simulink model "project_589"  (R2020b)
settings: Solver=VariableStepAuto  StartTime=0.0  StopTime=2  RelTol=1e-3
libraries: powerlib x25, powerlib_meascontrol x8, simulink x7, re_lib x2, fillib x1
(part 1 of 2)
settings Model: Creator=mcapuano  LastModifiedBy=mcapuano
settings DebuggingCC: IgnoredZcDiagnostic=none

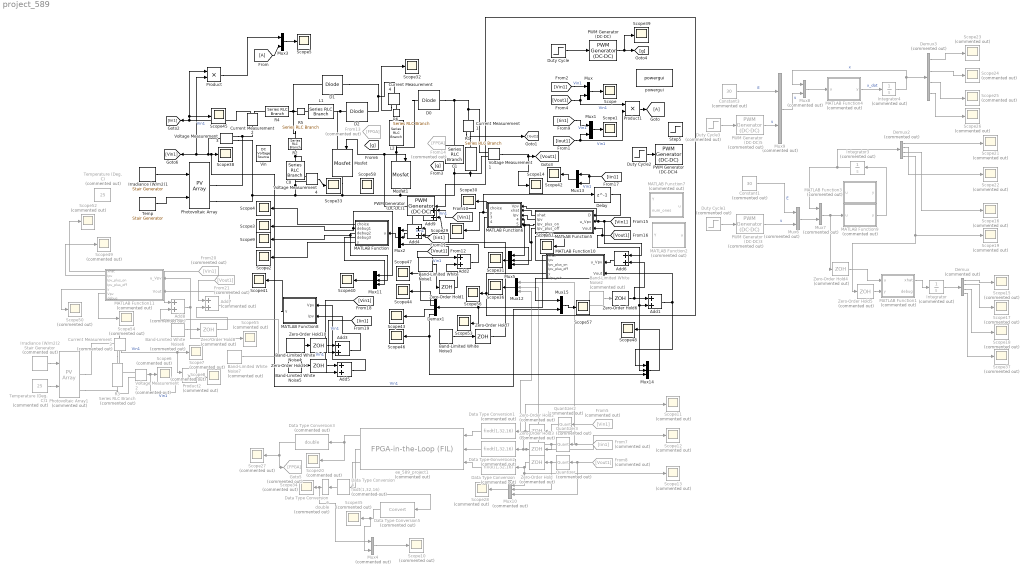
== system project_589 ==
  " Temp" : powerlib_meascontrol/Pulse & Signal Generators/Stair Generator  t=[0 .5 1 1.5]  e=[25 25 35 45]  Ts=15e-6
  Add{1..6,9} (7 alike) : Sum
  Add7 : Sum  Commented=on
  Add8 : Sum  Commented=on
  Band-Limited White Noise{1,3..5} (4 alike) : simulink/Sources/Band-Limited White Noise  Cov=[.0001]  Ts=1e-3  seed=[23341]
  Band-Limited White Noise2 : simulink/Sources/Band-Limited White Noise  Commented=on  Cov=[.00001]  Ts=15e-6  seed=[23341]
  Band-Limited White Noise6 : simulink/Sources/Band-Limited White Noise  Commented=on  Cov=[.0000001]  Ts=1e-6  seed=[23341]
  Band-Limited White Noise7 : simulink/Sources/Band-Limited White Noise  Commented=on  Cov=[.0000001]  Ts=15e-6  seed=[23341]
  C0 : powerlib/Elements/Series RLC Branch  LConnTagsString=__new0  RConnTagsString=__new0  BranchType=C  Resistance=1e-4  Inductance=200e-6  SetiL0=off  InitialCurrent=0  Capacitance=260e-6  Setx0=on  InitialVoltage=0  Measurements=None
  C1 : powerlib/Elements/Series RLC Branch  LConnTagsString=__new0  RConnTagsString=__new0  BranchType=C  Resistance=1e-4  Inductance=200e-6  SetiL0=off  InitialCurrent=0  Capacitance=260e-6  Setx0=on  InitialVoltage=0  Measurements=None
  Constant1 : Constant  Commented=on  Value=30
  Constant3 : Constant  Commented=on  Value=30
  Current Measurement1 : powerlib/Measurements/Current Measurement  PhasorSimulation=off  OutputType=Complex  PSBequivalent=0
  Current Measurement2 : powerlib/Measurements/Current Measurement  PhasorSimulation=off  OutputType=Complex  PSBequivalent=0
  Current Measurement3 : powerlib/Measurements/Current Measurement  Commented=on  PhasorSimulation=off  OutputType=Complex  PSBequivalent=0
  Current Measurement4 : powerlib/Measurements/Current Measurement  PhasorSimulation=off  OutputType=Complex  PSBequivalent=0
  D0 : powerlib/Power Electronics/Diode  Ron=1e-3  Lon=0  Vf=0  IC=0  UseSnubber=off  Rs=inf  Cs=inf  Measurements=off
  D1 : powerlib/Power Electronics/Diode  Ron=1e-3  Lon=0  Vf=0  IC=0  UseSnubber=off  Rs=inf  Cs=inf  Measurements=off
  D2 : powerlib/Power Electronics/Diode  Ron=1e-3  Lon=0  Vf=0  IC=0  UseSnubber=off  Rs=inf  Cs=inf  Measurements=off
  Data Type Conversion{,1..2,4} (4 alike) : DataTypeConversion  Commented=on  OutDataTypeStr=fixdt(1,32,16)
  Data Type Conversion3 : DataTypeConversion  Commented=on  OutDataTypeStr=double
  Data Type Conversion5 : DataTypeConversion  Commented=on
  Data Type Conversion6 : DataTypeConversion  Commented=on  OutDataTypeStr=double
  Delay : Delay  DelayLength=1  InitialCondition=0  SampleTime=15e-6
  Demux : Demux  Commented=on
  Demux1 : Demux
  Demux2 : Demux  Commented=on
  Demux3 : Demux  Commented=on
  Duty Cycle : Step  Time=.5  Before=.5  After=.5  SampleTime=0
  Duty Cycle1 : Step  Commented=on  Time=.5  Before=.5  After=.5  SampleTime=0
  Duty Cycle2 : Step  Time=.1  Before=.3  After=.5  SampleTime=0
  Duty Cycle3 : Step  Commented=on  Time=.5  Before=.5  After=.5  SampleTime=0
  From13 : From  Commented=on  GotoTag=FPGA
  From14 : From  Commented=on  GotoTag=FPGA
  From20 : From  Commented=on  GotoTag=Vin1
  From21 : From  Commented=on  GotoTag=Vout1
  From5 : From  Commented=on  GotoTag=Vin1
  From7 : From  Commented=on  GotoTag=Iin1
  From8 : From  Commented=on  GotoTag=Vout1
  Goto5 : Goto  Commented=on  GotoTag=FPGA
  Integrator : Integrator  Commented=on  InitialCondition=[0 0 0 0]
  Integrator3 : Integrator  Commented=on  InitialCondition=[0 0 0 0]
  Integrator4 : Integrator  Commented=on  InitialCondition=zeros(4,1)
  Irradiance (W/m2)1 : powerlib_meascontrol/Pulse & Signal Generators/Stair Generator  t=[0 .5]  e=[800 1000]  Ts=15e-6
  Irradiance (W/m2)2 : powerlib_meascontrol/Pulse & Signal Generators/Stair Generator  Commented=on  t=[0, 0.5, 1, 1.5, 2]  e=[0.5,0.7, 0.8, 0.6, 0.2]*1000  Ts=0.0001
  L1 : powerlib/Elements/Series RLC Branch  LConnTagsString=__new0  RConnTagsString=__new0  BranchType=L  Resistance=1e-4  Inductance=3e-3  SetiL0=on  InitialCurrent=0  Capacitance=30e-6  Setx0=off  InitialVoltage=150  Measurements=None
  L2 : powerlib/Elements/Series RLC Branch  LConnTagsString=__new0  RConnTagsString=__new0  BranchType=L  Resistance=1e-4  Inductance=3e-3  SetiL0=on  InitialCurrent=0  Capacitance=30e-6  Setx0=off  InitialVoltage=150  Measurements=None
  MATLAB Function : MATLAB Function  TreatAsAtomicUnit=on  SystemSampleTime=15e-6
  MATLAB Function1 : MATLAB Function  Commented=on  TreatAsAtomicUnit=on
  MATLAB Function10 : MATLAB Function  TreatAsAtomicUnit=on  SystemSampleTime=15e-6
  MATLAB Function11 : MATLAB Function  Commented=on  TreatAsAtomicUnit=on  SystemSampleTime=15e-6
  MATLAB Function2 : MATLAB Function  Commented=on  TreatAsAtomicUnit=on  SystemSampleTime=15e-6
  MATLAB Function3 : MATLAB Function  Commented=on  TreatAsAtomicUnit=on
  MATLAB Function4 : MATLAB Function  Commented=on  TreatAsAtomicUnit=on
  MATLAB Function5 : MATLAB Function  TreatAsAtomicUnit=on  SystemSampleTime=15e-6
  MATLAB Function6 : MATLAB Function  TreatAsAtomicUnit=on  SystemSampleTime=15e-6
  MATLAB Function7 : MATLAB Function  Commented=on  TreatAsAtomicUnit=on  SystemSampleTime=15e-6
  MATLAB Function8 : MATLAB Function  TreatAsAtomicUnit=on  SystemSampleTime=15e-6
  MATLAB Function9 : MATLAB Function  Commented=on  TreatAsAtomicUnit=on
  Mosfet : powerlib/Power Electronics/Mosfet  Ron=1e-3  Lon=0  Rd=1e-3  Vfd=0  IC=0  Rs=1e6  Cs=inf  Measurements=off
  Mosfet1 : powerlib/Power Electronics/Mosfet  Ron=1e-3  Lon=0  Rd=1e-3  Vfd=0  IC=0  Rs=1e6  Cs=inf  Measurements=off
  Mux{,1,3,13,15} (5 alike) : Mux  Inputs=2
  Mux10 : Mux  Commented=on  Inputs=3
  Mux{2,5,11..12,14} (5 alike) : Mux  Inputs=3
  Mux{4,6..9} (5 alike) : Mux  Commented=on  Inputs=2
  PWM Generator (DC-DC) : powerlib_meascontrol/Pulse & Signal Generators/PWM Generator (DC-DC)  Fsw=66.67e3  Ts=0
  PWM Generator (DC-DC)1 : powerlib_meascontrol/Pulse & Signal Generators/PWM Generator (DC-DC)  Fsw=66.67e3  Ts=0
  PWM Generator (DC-DC)3 : powerlib_meascontrol/Pulse & Signal Generators/PWM Generator (DC-DC)  Commented=on  Fsw=66.67e3  Ts=0
  PWM Generator (DC-DC)4 : powerlib_meascontrol/Pulse & Signal Generators/PWM Generator (DC-DC)  Fsw=66.67e3  Ts=0
  PWM Generator (DC-DC)5 : powerlib_meascontrol/Pulse & Signal Generators/PWM Generator (DC-DC)  Commented=on  Fsw=66.67e3  Ts=0
  Photovoltaic Array : re_lib/Solar/PV Array  Npar=1  Nser=1  PlotType=array @ 25 deg.C & specified irradiances  S_vec=[600 800 1000 1200]  Temp_C_vec=[25 50 75 100]  ModuleName=Kyocera Solar KC200GT  PlotWhenSelected=off  Pm=200.143  Ncell=54  Voc=32.9  Isc=8.21  Vm=26.3  Im=7.61  beta_Voc_pc=-0.355  alpha_Isc_pc=0.06  beta_Voc=-0.11679  alpha_Isc=0.004926  IL=8.2288  I0=2.3234e-10  nI=0.97734  Rsh=150.6844  Rs=0.34484  RobustModel=off  RobustCellTemperature=313.3991  BAL=on  Tc=1e-6  Tfilter=5e-5
      settings: AttributesFormatString=|
      | %<ModuleName>
      | %<Nser>-module string
      | %<Npar> parallel strings
  Photovoltaic Array1 : re_lib/Solar/PV Array  Commented=on  Npar=1  Nser=1  PlotType=one module @ 25 deg.C & specified irradiances  S_vec=[800]  Temp_C_vec=[ 50 ]  ModuleName=Kyocera Solar KC200GT  PlotWhenSelected=off  Pm=200.143  Ncell=54  Voc=32.9  Isc=8.21  Vm=26.3  Im=7.61  beta_Voc_pc=-0.355  alpha_Isc_pc=0.06  beta_Voc=-0.11679  alpha_Isc=0.004926  IL=8.2288  I0=2.3234e-10  nI=0.97734  Rsh=150.6844  Rs=0.34484  RobustModel=off  RobustCellTemperature=313.3991  BAL=on  Tc=1e-6  Tfilter=5e-5
      settings: AttributesFormatString=|
      | %<ModuleName>
      | %<Nser>-module string
      | %<Npar> parallel strings
  Product : Product
  Product1 : Product
  Product2 : Product  Commented=on
  Quantizer : Quantizer  Commented=on  QuantizationInterval=15e-6
  Quantizer2 : Quantizer  Commented=on  QuantizationInterval=15e-6
  Quantizer3 : Quantizer  Commented=on  QuantizationInterval=15e-6
  R1 : powerlib/Elements/Series RLC Branch  LConnTagsString=__new0  RConnTagsString=__new0  BranchType=R  Resistance=100  Inductance=200e-6  SetiL0=off  InitialCurrent=0  Capacitance=400e-6  Setx0=off  InitialVoltage=0  Measurements=None
  R2 : powerlib/Elements/Series RLC Branch  LConnTagsString=__new0  RConnTagsString=__new0  BranchType=R  Resistance=.01  Inductance=200e-6  SetiL0=off  InitialCurrent=0  Capacitance=400e-6  Setx0=off  InitialVoltage=0  Measurements=None
  R3 : powerlib/Elements/Series RLC Branch  Commented=on  LConnTagsString=__new0  RConnTagsString=__new0  BranchType=R  Resistance=1  Inductance=200e-6  SetiL0=off  InitialCurrent=0  Capacitance=400e-6  Setx0=off  InitialVoltage=0  Measurements=None
  R4 : powerlib/Elements/Series RLC Branch  LConnTagsString=__new0  RConnTagsString=__new0  BranchType=R  Resistance=.1  Inductance=200e-6  SetiL0=off  InitialCurrent=0  Capacitance=400e-6  Setx0=off  InitialVoltage=0  Measurements=None
  R5 : powerlib/Elements/Series RLC Branch  LConnTagsString=__new0  RConnTagsString=__new0  BranchType=R  Resistance=.0000001  Inductance=200e-6  SetiL0=off  InitialCurrent=0  Capacitance=400e-6  Setx0=off  InitialVoltage=0  Measurements=None
  R6 : powerlib/Elements/Series RLC Branch  LConnTagsString=__new0  RConnTagsString=__new0  BranchType=R  Resistance=.0000001  Inductance=200e-6  SetiL0=off  InitialCurrent=0  Capacitance=400e-6  Setx0=off  InitialVoltage=0  Measurements=None
  Scope{,1..5,9,14,29..33,36,38..48,51,53,56..58} (30 alike) : Scope
  Scope{6..8,10..13,15..28,34..35,37,49..50,52,54..55} (29 alike) : Scope  Commented=on
  Step5 : Step  Time=.1  Before=.1  After=.6  SampleTime=0
  Temperature (Deg. C) : Constant  Commented=on  Value=25
  Temperature (Deg. C)1 : Constant  Commented=on  Value=25
  Vin : powerlib/Electrical Sources/DC Voltage Source  Amplitude=30  Measurements=None
  Voltage Measurement1 : powerlib/Measurements/Voltage Measurement  PhasorSimulation=off  OutputType=Complex  PSBequivalent=0
  Voltage Measurement2 : powerlib/Measurements/Voltage Measurement  Commented=on  PhasorSimulation=off  OutputType=Complex  PSBequivalent=0
  Voltage Measurement3 : powerlib/Measurements/Voltage Measurement  PhasorSimulation=off  OutputType=Complex  PSBequivalent=0
  Voltage Measurement4 : powerlib/Measurements/Voltage Measurement  PhasorSimulation=off  OutputType=Complex  PSBequivalent=0
  Zero-Order Hold : ZeroOrderHold  Commented=on  SampleTime=200e-9
  Zero-Order Hold{1,6..7,10..11} (5 alike) : ZeroOrderHold  SampleTime=15e-6
  Zero-Order Hold2 : ZeroOrderHold  Commented=on  SampleTime=200e-9
  Zero-Order Hold3 : ZeroOrderHold  Commented=on  SampleTime=200e-9
  Zero-Order Hold4 : ZeroOrderHold  Commented=on  SampleTime=15e-6
  Zero-Order Hold5 : ZeroOrderHold  Commented=on  SampleTime=15e-6
  Zero-Order Hold8 : ZeroOrderHold  Commented=on  SampleTime=15e-6
  ee_589_project1 : fillib/FPGA-in-the-Loop (FIL)  Commented=on  ForceInterfaceUpdate=0.91338
      settings: SourceProductBaseCode=ES,HD
  powergui : powerlib/powergui  Priority=1  SimulationMode=Continuous  SampleTime=50e-6  frequency=60  Iterations=50  frequencyindice=0  Pbase=100e6  ErrMax=1e-4  UnitsV=kV  UnitsW=MW  buscounter=0  FunctionMessages=off  echomessages=off  EnableUseOfTLC=off  CurrentSourceSwitches=off  DisableSnubberDevices=off  DisableRonSwitches=off  DisableVfSwitches=off  DisplayEquations=off  AutomaticDiscreteSolvers=off  SolverType=Tustin/Backward Euler (TBE)  Interpol=off  ExternalGateDelay=off  methode=off  Ts=100  x0status=blocks  SPID=on  SwTol=0  HookPort=off  NonlinearTolerance=1e-4  nMaxIteration=100  ContinueOnMaxIteration=off  RestoreLinks=warning  ResistiveCurrentMeasurement=off  Frange=[0:2:500]  Ylog=off  Xlog=on  ShowGrid=off  save=off  variable=ZData  structure=0  ZoomFFT=off  StartTime=0.0  cycles=1  DisplayStyle=1  fundamental=60  FreqAxis=off  MaxFrequency=1000  frequencyindicesteady=1  RmsSteady=1  display=off
  wires:
  Duty Cycle/1 -> PWM Generator (DC-DC)/1
  PWM Generator (DC-DC)/1 -> Scope39/1, [g]
  Current Measurement1/1 -> [Iout1]
  Mux1/1 -> Scope1/1
  [Iout1] -> Product1/2, Mux1/2  "Vin1"
  [Iin1] -> Mux1/1  "Vin1"
  [Vin1] -> Mux/1  "Vin1"
  Mux/1 -> Scope/1
  [Vout1] -> Mux/2, Product1/1  "Vin1"
  Mux2/1 -> MATLAB Function/1(u)
  MATLAB Function/2(debug1) -> Scope3/1, Mux11/1
  MATLAB Function/1(choice) -> Scope4/1
  Voltage Measurement3/1 -> Product/2, [Vin1], Mux15/2, Scope38/1  "Vin1"
  Product/1 -> Mux3/1
  Current Measurement2/1 -> Scope45/1, Product/1, [Iin1]  "Vin1"
  Irradiance (W/m2)1/1 -> Photovoltaic Array/1
  Mux3/1 -> Scope5/1
  [A] -> Mux3/2
  Product1/1 -> [A]
  Temperature (Deg. C)1/1 -> Photovoltaic Array1/2
  Irradiance (W/m2)2/1 -> Photovoltaic Array1/1
  Voltage Measurement2/1 -> Product2/2, Scope6/1  "Vin1"
  Current Measurement3/1 -> Scope7/1, Product2/1  "Vin1"
  Product2/1 -> Scope8/1
  Constant1/1 -> Mux6/1  "E"
  Mux6/1 -> Mux7/2
  Mux7/1 -> MATLAB Function9/1(u), Zero-Order Hold4/1
  Demux2/3 -> Scope16/1
  Integrator3/1 -> Demux2/1, Mux7/1
  Demux2/2 -> Scope22/1
  Demux2/4 -> Scope19/1, Zero-Order Hold5/1
  Demux2/1 -> Scope21/1
  PWM Generator (DC-DC)3/1 -> Mux6/2  "u"
  Duty Cycle1/1 -> PWM Generator (DC-DC)3/1
  Integrator4/1 -> Mux8/1, Demux3/1  "x"
  Constant3/1 -> Mux9/1  "E"
  Mux9/1 -> Mux8/2  "u"
  MATLAB Function4/1(y) -> Integrator4/1  "x_dot"
  Demux3/2 -> Scope24/1
  Demux3/1 -> Scope23/1
  Mux8/1 -> MATLAB Function4/1(u)
  Demux3/3 -> Scope25/1
  Demux3/4 -> Scope26/1
  Duty Cycle2/1 -> PWM Generator (DC-DC)4/1
  Mux10/1 -> Scope28/1
  Quantizer/1 -> Mux10/2, Zero-Order Hold/1
  Zero-Order Hold/1 -> Mux10/1, Scope13/1, Data Type Conversion/1
  Current Measurement4/1 -> Scope32/1
  Data Type Conversion2/1 -> ee_589_project1/2
  Data Type Conversion1/1 -> ee_589_project1/1
  Zero-Order Hold2/1 -> Scope11/1, Data Type Conversion1/1
  Zero-Order Hold3/1 -> Data Type Conversion2/1, Mux12/3, Scope12/1
  Quantizer3/1 -> Mux12/2, Zero-Order Hold3/1
  Quantizer2/1 -> Zero-Order Hold2/1
  From5/1 -> Quantizer2/1
  From7/1 -> Mux12/1, Quantizer3/1
  From8/1 -> Mux10/3, Quantizer/1
  Data Type Conversion5/1 -> Mux4/2, Scope35/1
  ee_589_project1/3 -> Data Type Conversion5/1
  Mux12/1 -> Scope36/1
  Data Type Conversion4/1 -> Data Type Conversion6/1
  Data Type Conversion3/1 -> Goto5/1, Scope27/1
  ee_589_project1/1 -> Data Type Conversion3/1, Scope20/1
  ee_589_project1/2 -> Data Type Conversion4/1
  Data Type Conversion6/1 -> Mux4/1, Scope34/1
  Data Type Conversion/1 -> ee_589_project1/3
  MATLAB Function/3(debug2) -> Mux11/2, Scope9/1
  Mux4/1 -> Scope10/1
  Demux/1 -> Scope15/1
  Demux/2 -> Scope17/1
  Demux/3 -> Scope18/1
  Demux/4 -> Scope37/1
  MATLAB Function1/1(xhat) -> Integrator/1
  Integrator/1 -> Demux/1
  Zero-Order Hold4/1 -> MATLAB Function1/1(u)
  Zero-Order Hold5/1 -> MATLAB Function1/2(y)
  MATLAB Function/5(y) -> Scope2/1
  [Vin1] -> Add6/1, MATLAB Function6/1(Vpv), MATLAB Function5/2(u_Vpv)
  [Vout1] -> Mux14/2, Add1/2, MATLAB Function5/3(Vout)
  MATLAB Function5/1(xhat) -> MATLAB Function6/2(xhat)
  MATLAB Function5/3(Ipv_plus_on) -> Mux5/1, MATLAB Function6/4(Ipv_plus_on)
  MATLAB Function5/4(Ipv_plus_off) -> Mux5/2, MATLAB Function6/5(Ipv_plus_off)
  MATLAB Function6/2(y) -> Delay/1, Scope29/1
  MATLAB Function6/1(choice) -> Scope30/1
  Mux5/1 -> Scope31/1
  Mux11/1 -> Scope40/1
  MATLAB Function/4(debug3) -> Mux11/3
  Mux13/1 -> Scope42/1
  [Iin1] -> Mux13/2, Mux13/1  "Vin1"
  Demux1/1 -> Scope47/1
  Demux1/2 -> Scope44/1
  Demux1/3 -> Scope43/1
  Demux1/4 -> Mux14/3, Scope46/1
  MATLAB Function6/3(debug1) -> Mux5/3
  MATLAB Function5/2(Ipv) -> MATLAB Function6/3(Ipv)
  MATLAB Function8/1(Y) -> Scope41/1
  Duty Cycle3/1 -> PWM Generator (DC-DC)5/1
  PWM Generator (DC-DC)5/1 -> Mux9/2  "u"
  MATLAB Function9/1(y) -> Integrator3/1
  Voltage Measurement4/1 -> Scope33/1
  Delay/1 -> MATLAB Function5/1(D)
  " Temp"/1 -> Photovoltaic Array/2
  Voltage Measurement1/1 -> Scope14/1, [Vout1]
  Band-Limited White Noise2/1 -> Zero-Order Hold6/1
  Zero-Order Hold6/1 -> Add6/2, Add1/1
  Add1/1 -> Mux14/1, MATLAB Function10/2(Vout)
  Zero-Order Hold1/1 -> Add2/2
  [Vout1] -> Add2/1  "Vin1"
  Add2/1 -> Mux2/3
  Band-Limited White Noise1/1 -> Zero-Order Hold1/1
  Add4/1 -> Mux2/2
  [Iin1] -> Add4/1  "Vin1"
  [Iin1] -> Add3/2  "Vin1"
  [Vin1] -> Add5/2  "Vin1"
  Add5/1 -> MATLAB Function8/1(Vpv)
  Add3/1 -> MATLAB Function8/2(Ipv)
  Zero-Order Hold7/1 -> Add4/2, Add9/2
  Band-Limited White Noise3/1 -> Zero-Order Hold7/1
  Mux14/1 -> Scope48/1
  Add6/1 -> MATLAB Function10/1(u_Vpv)
  MATLAB Function11/2(Ipv) -> Scope49/1
  MATLAB Function10/2(Ipv) -> Scope51/1
  MATLAB Function11/1(xhat) -> Scope52/1
  MATLAB Function10/1(xhat) -> Scope53/1, Demux1/1
  MATLAB Function11/6(Vpv) -> Scope54/1
  MATLAB Function10/5(y) -> PWM Generator (DC-DC)1/1, Scope56/1
  MATLAB Function11/5(y) -> Scope50/1
  Band-Limited White Noise6/1 -> Zero-Order Hold8/1
  Zero-Order Hold8/1 -> Add7/2
  From21/1 -> Add7/1
  Add7/1 -> MATLAB Function11/2(Vout)
  From20/1 -> Add8/1
  Add8/1 -> MATLAB Function11/1(u_Vpv), Scope55/1
  Band-Limited White Noise7/1 -> Add8/2
  Band-Limited White Noise4/1 -> Zero-Order Hold10/1
  Zero-Order Hold10/1 -> Add3/1
  Band-Limited White Noise5/1 -> Zero-Order Hold11/1
  Zero-Order Hold11/1 -> Add5/1
  [Vin1] -> Add9/1  "Vin1"
  Add9/1 -> Mux2/1
  PWM Generator (DC-DC)1/1 -> Mosfet/1, Mosfet1/1
  Mux15/1 -> Scope57/1
  MATLAB Function10/6(Vpv_out) -> Mux15/1
  connections:
  D0/RConn1 -- C1/LConn1 -- Current Measurement1/LConn1 -- Voltage Measurement1/LConn1
  R2/LConn1 -- R5/LConn1 -- R4/RConn1 -- D1/LConn1
  C1/RConn1 -- Mosfet/RConn1 -- Voltage Measurement3/LConn2 -- Photovoltaic Array/RConn2 -- Voltage Measurement4/LConn2 -- C0/RConn1 -- Mosfet1/RConn1 -- Voltage Measurement1/LConn2 -- R1/RConn1
  Mosfet/LConn1 -- L1/RConn1 -- D2/LConn1
  D1/RConn1 -- Current Measurement4/LConn1 -- D2/RConn1
  D0/LConn1 -- Mosfet1/LConn1 -- L2/RConn1
  Current Measurement1/RConn1 -- R1/LConn1
  R2/RConn1 -- Voltage Measurement4/LConn1 -- C0/LConn1
  Voltage Measurement3/LConn1 -- Current Measurement2/LConn1 -- Photovoltaic Array/RConn1
  Photovoltaic Array1/RConn1 -- Current Measurement3/LConn1 -- Voltage Measurement2/LConn1
  Photovoltaic Array1/RConn2 -- Voltage Measurement2/LConn2 -- R3/RConn1
  Current Measurement3/RConn1 -- R3/LConn1
  R4/LConn1 -- Current Measurement2/RConn1
  R5/RConn1 -- L1/LConn1
  R6/LConn1 -- Current Measurement4/RConn1
  R6/RConn1 -- L2/LConn1

== matlab function project_589/MATLAB Function9 ==
  data: u input; y output
function y = fcn(u)

X=u(1:4);
Vpv=u(5);
u=u(6);



% parameters:
%5/10/2021 u_ePDATED


Cpv=260e-6;
Cout=260e-6;
L1=3e-3;
L2=3e-3;
Rout=100;
Rpv = 1;
RL1 = 1;
RL2 = 1;

u_e = .5;

% Compact form
A=[(-1/(Cpv*Rpv)) (-1/(Cpv)) (-u_e/(Cpv)) 0 ;
    (1/(L1+L2) + L2*u_e/(L1*(L1+L2)))  (-RL1/(L1+L2) -RL1*L2*u_e/(L1*(L1+L2)))  (-RL2/(L1+L2) + RL2*u_e/(L1+L2)) (-1/(L1+L2) + u_e/(L1+L2));
    (1/(L1+L2) + L1*u_e/(L2*(L1+L2)))  (-RL1/(L1+L2) + RL1*u_e/(L1+L2)) (-RL2/(L1+L2)-RL2*L1*u_e/(L2*(L1+L2))) (-1/(L1+L2) + u_e/(L1+L2));
    0 0 (1/(Cout) - u_e/(Cout)) (-1/(Rout*Cout))];

%VCpv = (L2*RL1*Rout*Vpv*u_e^2 - 2*L2*RL1*Rout*Vpv*u_e + L1*RL1*RL2*Vpv + L2*RL1*RL2*Vpv + L2*RL1*Rout*Vpv)/(L1*RL1*RL2 + L2*RL1*RL2 + L2*RL1*Rout + L2*RL2*Rpv - L1*Rout*Rpv + L2*Rout*Rpv + L2*RL1*Rout*u_e^2 + L2*RL1*Rpv*u_e^2 - L1*Rout*Rpv*u_e^2 + L2*Rout*Rpv*u_e^2 - 2*L2*RL1*Rout*u_e + L1*RL1*Rpv*u_e + L1*RL2*Rpv*u_e + 2*L1*Rout*Rpv*u_e - 2*L2*Rout*Rpv*u_e);
%IL1 = (Vpv*(L2*RL2 - L1*Rout + L2*Rout + L1*RL2*u_e + 2*L1*Rout*u_e - 2*L2*Rout*u_e - L1*Rout*u_e^2 + L2*Rout*u_e^2))/(L1*RL1*RL2 + L2*RL1*RL2 + L2*RL1*Rout + L2*RL2*Rpv - L1*Rout*Rpv + L2*Rout*Rpv + L2*RL1*Rout*u_e^2 + L2*RL1*Rpv*u_e^2 - L1*Rout*Rpv*u_e^2 + L2*Rout*Rpv*u_e^2 - 2*L2*RL1*Rout*u_e + L1*RL1*Rpv*u_e + L1*RL2*Rpv*u_e + 2*L1*Rout*Rpv*u_e - 2*L2*Rout*Rpv*u_e);
%IL2 = (RL1*Vpv*(L1 + L2*u_e))/(L1*RL1*RL2 + L2*RL1*RL2 + L2*RL1*Rout + L2*RL2*Rpv - L1*Rout*Rpv + L2*Rout*Rpv + L2*RL1*Rout*u_e^2 + L2*RL1*Rpv*u_e^2 - L1*Rout*Rpv*u_e^2 + L2*Rout*Rpv*u_e^2 - 2*L2*RL1*Rout*u_e + L1*RL1*Rpv*u_e + L1*RL2*Rpv*u_e + 2*L1*Rout*Rpv*u_e - 2*L2*Rout*Rpv*u_e);
%VCout = -(RL1*Rout*Vpv*(L1 + L2*u_e)*(u_e - 1))/(L1*RL1*RL2 + L2*RL1*RL2 + L2*RL1*Rout + L2*RL2*Rpv - L1*Rout*Rpv + L2*Rout*Rpv + L2*RL1*Rout*u_e^2 + L2*RL1*Rpv*u_e^2 - L1*Rout*Rpv*u_e^2 + L2*Rout*Rpv*u_e^2 - 2*L2*RL1*Rout*u_e + L1*RL1*Rpv*u_e + L1*RL2*Rpv*u_e + 2*L1*Rout*Rpv*u_e - 2*L2*Rout*Rpv*u_e);

VCpv = (L2*RL1*Rout*Vpv*u_e^2 - 2*L2*RL1*Rout*Vpv*u_e + L1*RL1*RL2*Vpv + L2*RL1*RL2*Vpv + L2*RL1*Rout*Vpv)/(L1*RL1*RL2 + L2*RL1*RL2 + L2*RL1*Rout + L2*RL2*Rpv - L1*Rout*Rpv + L2*Rout*Rpv + L2*RL1*Rout*u_e^2 + L2*RL1*Rpv*u_e^2 - L1*Rout*Rpv*u_e^2 + L2*Rout*Rpv*u_e^2 - 2*L2*RL1*Rout*u_e + L1*RL1*Rpv*u_e + L1*RL2*Rpv*u_e + 2*L1*Rout*Rpv*u_e - 2*L2*Rout*Rpv*u_e);
IL1 = (Vpv*(L2*RL2 - L1*Rout + L2*Rout + L1*RL2*u_e + 2*L1*Rout*u_e - 2*L2*Rout*u_e - L1*Rout*u_e^2 + L2*Rout*u_e^2))/(L1*RL1*RL2 + L2*RL1*RL2 + L2*RL1*Rout + L2*RL2*Rpv - L1*Rout*Rpv + L2*Rout*Rpv + L2*RL1*Rout*u_e^2 + L2*RL1*Rpv*u_e^2 - L1*Rout*Rpv*u_e^2 + L2*Rout*Rpv*u_e^2 - 2*L2*RL1*Rout*u_e + L1*RL1*Rpv*u_e + L1*RL2*Rpv*u_e + 2*L1*Rout*Rpv*u_e - 2*L2*Rout*Rpv*u_e);
IL2 =  (RL1*Vpv*(L1 + L2*u_e))/(L1*RL1*RL2 + L2*RL1*RL2 + L2*RL1*Rout + L2*RL2*Rpv - L1*Rout*Rpv + L2*Rout*Rpv + L2*RL1*Rout*u_e^2 + L2*RL1*Rpv*u_e^2 - L1*Rout*Rpv*u_e^2 + L2*Rout*Rpv*u_e^2 - 2*L2*RL1*Rout*u_e + L1*RL1*Rpv*u_e + L1*RL2*Rpv*u_e + 2*L1*Rout*Rpv*u_e - 2*L2*Rout*Rpv*u_e);
VCout =  -(RL1*Rout*Vpv*(L1 + L2*u_e)*(u_e - 1))/(L1*RL1*RL2 + L2*RL1*RL2 + L2*RL1*Rout + L2*RL2*Rpv - L1*Rout*Rpv + L2*Rout*Rpv + L2*RL1*Rout*u_e^2 + L2*RL1*Rpv*u_e^2 - L1*Rout*Rpv*u_e^2 + L2*Rout*Rpv*u_e^2 - 2*L2*RL1*Rout*u_e + L1*RL1*Rpv*u_e + L1*RL2*Rpv*u_e + 2*L1*Rout*Rpv*u_e - 2*L2*Rout*Rpv*u_e);
 
B=[ -IL2/Cpv;
    L2*VCpv/(L1*(L1+L2))-RL1*L2*IL1/(L1*(L1+L2))+RL2*IL2/(L1+L2)+VCout/(L1+L2);
    L1*VCpv/(L2*(L1+L2))+RL1*IL1/(L1+L2)-RL2*L1*IL2/(L2*(L1+L2))+VCout/(L1+L2);
     -IL2/Cout];


% B = [1/(Cpv*Rpv);
%     0;
%     0;
%     0];

%u = Vpv;

y = A*X+B*u;

== matlab function project_589/MATLAB Function10 ==
  data: xhat output; u_Vpv input; Vout input; Ipv output; Ipv_plus_on output; Ipv_plus_off output; y output; Vpv_out output
function [xhat, Ipv, Ipv_plus_on, Ipv_plus_off, y, Vpv_out]  = fcn(u_Vpv, Vout)
%Kalman filter design using Small Signal Model of Circuit

%The purpose of this module is to approximate Ipv and Vpv so that a sensor
%is not needed for those variables, it also functions to remove noise and
%could possibly replace the MCP module using its own predictions

%Existing Model assumes Constant Vpv with added series resistor so that
% Ipv = (Vpv - Vcpv)/Rpv
%Also assumes L1 = L2

%Existing state variables: IL1 IL2 Vo Vcpv

%define circuit parameters 


Cpv=260e-6;
Cout=260e-6;
L1=3e-3;
L2=3e-3;
Rout=100;
Rpv = .1;
RL1 = .0000001;
RL2 = .0000001;

persistent Est_Vpv;
if isempty(Est_Vpv)
    Est_Vpv = 0;
end
persistent DC;
if isempty(DC)
    DC = 0;
end
Vpv = u_Vpv;
y = Vout;
u = u_Vpv;

Ts = 15e-6;
% Continuous Time Small Signal State Space
%Aol = [0.943784461257301,-0.0559330122345799,-0.0279395312339836,5.29606701473712e-05;0.00363447688363775,0.996152021590196,-0.00131615408875196,-0.00124644633684318;0.00363447688363775,-0.00135110080726459,0.996186968308708,-0.00124644633684318;5.29606701473712e-05,-1.90030480999995e-05,0.0287831492829427,0.999405251934562];
Ac =[(-1/(Cpv*Rpv)) (-1/(Cpv)) (-DC/(Cpv)) 0 ;
    (1/(L1+L2) + L2*DC/(L1*(L1+L2)))  (-RL1/(L1+L2) -RL1*L2*DC/(L1*(L1+L2)))  (-RL2/(L1+L2) + RL2*DC/(L1+L2)) (-1/(L1+L2) + DC/(L1+L2));
    (1/(L1+L2) + L1*DC/(L2*(L1+L2)))  (-RL1/(L1+L2) + RL1*DC/(L1+L2)) (-RL2/(L1+L2)-RL2*L1*DC/(L2*(L1+L2))) (-1/(L1+L2) + DC/(L1+L2));
    0 0 (1/(Cout) - DC/(Cout)) (-1/(Rout*Cout))];
Bc = [1/(Cpv*Rpv);
    0;
    0;
    0];
 Cc = [0 0 0 1];
 
 Dc = zeros(size(Cc,1), size(Bc,2));
 
 %discretize my state space model using ZOH method
 Aol = eye(4) + Ac*Ts;
 Bol = Bc*Ts;
 Col = Cc;
 Dol = Dc;
 
 
%Bol = [0.0560566260169120;0.000105941817191590;0.000105941817191590;1.02384484238660e-06];

%Col = [0,0,0,1];

%Dol = 0;
 %Design the Observer System:
 

 %covar matricies, process q, measurement r -- must be positive numbers
 Qcov = diag(.000000001*ones(1,4)); %modify the numbers to change how it filters noise
 Rcov = diag(.01*ones(1,1)); %modify the numbers to change how it filters noise
 

persistent xhat_t_1; %previous xhat Sample
if isempty(xhat_t_1)
    xhat_t_1 = [.1; .1; .1; .1];
end

persistent P_t_1;
if isempty(P_t_1)
    P_t_1 = [.1 .1 .1 .1;
            .1 .1 .1 .1;
            .1 .1 .1 .1;
            .1 .1 .1 .1];
end


%prediction stage
xhat_pred = Aol*xhat_t_1+Bol*u;
P_pred = Aol*P_t_1*transpose(Aol)+ Qcov;

%update stage
y_update = y - Col*xhat_pred;
S_update = Col*P_pred*transpose(Col) + Rcov;
K_update = P_pred*transpose(Col)*(1/S_update);
xhat_update = xhat_pred + K_update*y_update;
P_update = (eye(4) - K_update*Col)*P_pred;

Est_Vpv =  xhat_update(4)*(1-DC)/(1+DC) + .35;
 Vpv_out = Est_Vpv;

%increase DC by .01:
DC = DC + .0001;
if(DC > 1)
    DC = 1;
end
Ac =[(-1/(Cpv*Rpv)) (-1/(Cpv)) (-DC/(Cpv)) 0 ;
    (1/(L1+L2) + L2*DC/(L1*(L1+L2)))  (-RL1/(L1+L2) -RL1*L2*DC/(L1*(L1+L2)))  (-RL2/(L1+L2) + RL2*DC/(L1+L2)) (-1/(L1+L2) + DC/(L1+L2));
    (1/(L1+L2) + L1*DC/(L2*(L1+L2)))  (-RL1/(L1+L2) + RL1*DC/(L1+L2)) (-RL2/(L1+L2)-RL2*L1*DC/(L2*(L1+L2))) (-1/(L1+L2) + DC/(L1+L2));
    0 0 (1/(Cout) - DC/(Cout)) (-1/(Rout*Cout))];
Aol_increase = eye(4) + Ac*Ts;
%predict 1 timestep ahead on
xhat_plus_on = Aol_increase*xhat_update + Bol*u;
Ipv_plus_on = (u - xhat_plus_on(1))/Rpv;
%decrease DC by .01
DC = DC - 2*.0001;
if(DC < 0) 
    DC = 0; end
Ac =[(-1/(Cpv*Rpv)) (-1/(Cpv)) (-DC/(Cpv)) 0 ;
    (1/(L1+L2) + L2*DC/(L1*(L1+L2)))  (-RL1/(L1+L2) -RL1*L2*DC/(L1*(L1+L2)))  (-RL2/(L1+L2) + RL2*DC/(L1+L2)) (-1/(L1+L2) + DC/(L1+L2));
    (1/(L1+L2) + L1*DC/(L2*(L1+L2)))  (-RL1/(L1+L2) + RL1*DC/(L1+L2)) (-RL2/(L1+L2)-RL2*L1*DC/(L2*(L1+L2))) (-1/(L1+L2) + DC/(L1+L2));
    0 0 (1/(Cout) - DC/(Cout)) (-1/(Rout*Cout))];
DC = DC + .0001;
Aol_decrease = eye(4) + Ac*Ts;
%predict 1 timestep ahead off
xhat_plus_off = Aol_decrease*xhat_update + Bol*u;
Ipv_plus_off = (u - xhat_plus_off(1))/Rpv;

%update function output and variables
P_t_1 = P_update;
xhat_t_1 = xhat_update;
xhat = xhat_update;
Ipv = (u - xhat(1))/Rpv;

%%%%%%%%%%%%%%%%%%%%%%%%%%%%%%%
if (Ipv > 10)
    Ipv = 1;
end



persistent Vpv_t_1; %previous Vpv Sample
if isempty(Vpv_t_1)
    Vpv_t_1 = 0;
end
persistent Ipv_t_1; %previous Ipv Sample
if isempty(Ipv_t_1)
    Ipv_t_1 = 0;
end
persistent Dpv_t_1; % Iref (output) value from what is now 2 timesteps ago
if isempty(Dpv_t_1)
    Dpv_t_1 = 0;
end
persistent Dpv;  %Previous / Most recent Iref (output) Calc
if isempty(Dpv)
    Dpv = 0;
end

Ts = 15e-6; %sample rate
L = 3e-3; %inductance


delta_V = Vpv - Vpv_t_1;
delta_I = Ipv - Ipv_t_1;
delta_D = Dpv - Dpv_t_1;


%fixed vs adaptive
scale_factor_C = 10; %increase for larger output increments/swings
 Z =.001; %fixed 
%Z = scale_factor_C * abs(delta_I * delta_D); %adaptive

% custom adaptive to fix issues with no change causing 0 step size
 adapZ = scale_factor_C * abs(delta_I * delta_D);
% if(adapZ > .1)
%     Z = .1;
% elseif(adapZ > .001)
%     Z = adapZ;
% else
%     Z = .001;
% end

Ipred_1 = Ipv_plus_on;
Ipred_0 = Ipv_plus_off;
%Ipred_1 = Ipv + 2*(Ts/L) * Vpv; %MPC prediction for switch = 1
%Ipred_0 = Ipv + (Ts/(2*L)* (Vpv - Vout)); %MPC prediction for switch = 0 

if delta_V == 0 %Inc. Cond. Algo to determine Iref
    if delta_I == 0 
        Iref = Dpv; choice = 0;
    else
        if delta_I > 0
            Iref = Dpv - Z; choice = 1;
        else
            Iref = Dpv + Z; choice = 2;
        end
    end
else
    if (Ipv + (delta_I/delta_V) * Vpv) == 0
        Iref = Dpv; choice = 3;
    else
        if (Ipv + (delta_I/delta_V) * Vpv) > 0
            Iref = Dpv - Z; choice = 4;
        else
            Iref = Dpv + Z; choice = 5;
        end
    end
end

G1 = abs(Iref - Ipred_1); %Optimize MPC by applying Iref
G0 = abs(Iref - Ipred_0);
if G1 < G0
    DC = DC + .0001;
else
    DC = DC - .0001;
end

if (DC < 0)
    DC = 0;
end
if (DC > 1)
    DC = 1;
end

if (Iref < 0)
    Iref = .001;
end
%test = Ipv + (delta_I/delta_V) * Vpv;
test =  delta_V;
%update static variables here:
Vpv_t_1 = Vpv; %previous Vpv Sample
Ipv_t_1 = Ipv; %previous Ipv Sample
Dpv_t_1 = Dpv; % Iref (output) value from what is now 2 timesteps ago
Dpv = Iref;  %Previous / Most recent Iref (output) Calc

y = DC;

%debug purposes:
debug1 = Iref;
debug2 = delta_I/delta_V;

== matlab function project_589/MATLAB Function11 ==
  data: xhat output; u_Vpv input; Vout input; Ipv output; Ipv_plus_on output; Ipv_plus_off output; y output; Vpv output; debug output
function [xhat, Ipv, Ipv_plus_on, Ipv_plus_off, y, Vpv, debug]  = fcn(u_Vpv, Vout)
%Kalman filter design using Small Signal Model of Circuit

%The purpose of this module is to approximate Ipv and Vpv so that a sensor
%is not needed for those variables, it also functions to remove noise and
%could possibly replace the MCP module using its own predictions

%Existing Model assumes Constant Vpv with added series resistor so that
% Ipv = (Vpv - Vcpv)/Rpv
%Also assumes L1 = L2

%Existing state variables: IL1 IL2 Vo Vcpv

%define circuit parameters 


Cpv=260e-6;
Cout=260e-6;
L1=3e-3;
L2=3e-3;
Rout=100;
Rpv = 1;
RL1 = 1;
RL2 = 1;
persistent DC;
if isempty(DC)
    DC = 0;
end

y = Vout;
u = u_Vpv;

Ts = 15e-6;
% Continuous Time Small Signal State Space
%Aol = [0.943784461257301,-0.0559330122345799,-0.0279395312339836,5.29606701473712e-05;0.00363447688363775,0.996152021590196,-0.00131615408875196,-0.00124644633684318;0.00363447688363775,-0.00135110080726459,0.996186968308708,-0.00124644633684318;5.29606701473712e-05,-1.90030480999995e-05,0.0287831492829427,0.999405251934562];
Ac =[(-1/(Cpv*Rpv)) (-1/(Cpv)) (-DC/(Cpv)) 0 ;
    (1/(L1+L2) + L2*DC/(L1*(L1+L2)))  (-RL1/(L1+L2) -RL1*L2*DC/(L1*(L1+L2)))  (-RL2/(L1+L2) + RL2*DC/(L1+L2)) (-1/(L1+L2) + DC/(L1+L2));
    (1/(L1+L2) + L1*DC/(L2*(L1+L2)))  (-RL1/(L1+L2) + RL1*DC/(L1+L2)) (-RL2/(L1+L2)-RL2*L1*DC/(L2*(L1+L2))) (-1/(L1+L2) + DC/(L1+L2));
    0 0 (1/(Cout) - DC/(Cout)) (-1/(Rout*Cout))];
Bc = [1/(Cpv*Rpv);
    0;
    0;
    0];
 Cc = [0 0 0 1];
 
 Dc = zeros(size(Cc,1), size(Bc,2));
 
 %discretize my state space model using ZOH method
 Aol = eye(4) + Ac*Ts;
 Bol = Bc*Ts;
 Col = Cc;
 Dol = Dc;
 
 
%Bol = [0.0560566260169120;0.000105941817191590;0.000105941817191590;1.02384484238660e-06];

%Col = [0,0,0,1];

%Dol = 0;
 %Design the Observer System:
 

 %covar matricies, process q, measurement r -- must be positive numbers
 Qcov = diag(1*ones(1,4)); %modify the numbers to change how it filters noise
 Rcov = diag(1*ones(1,1)); %modify the numbers to change how it filters noise
 
variance = 1;
persistent xhat_t_1; %previous xhat Sample
if isempty(xhat_t_1)
    xhat_t_1 = [.1; .1; .1; .1];
end

persistent P_t_1;
if isempty(P_t_1)
    P_t_1 = [.1 .1 .1 .1 ;
            .1 .1 .1 .1 ;
            .1 .1 .1 .1 ;
            .1 .1 .1 .1 ];
end


%prediction stage
xhat_pred = Aol*xhat_t_1+Bol*u;
P_pred = Aol*P_t_1*transpose(Aol)+ variance*Bol*transpose(Bol) + Qcov;

%update stage
y_update = y - Col*xhat_pred;
S_update = Col*P_pred*transpose(Col) + Rcov - variance;
K_update = P_pred*transpose(Col)*(1/S_update);
xhat_update = xhat_pred + K_update*y_update;
P_update = (eye(4) - K_update*Col)*P_pred;


    Ipv1 = xhat_update(2) + xhat_update(3) + Cpv*((xhat_update(1) - xhat_t_1(1)) / Ts); debug = 1;
 
    Ipv0 = xhat_update(2) + Cpv*((xhat_update(1) - xhat_t_1(1)) / Ts); debug = 0;

    Ipv = (Ipv1*DC + Ipv0*(1-DC));

    if(Ipv < 0)
        Ipv = 0;
    end
    
u = Ipv * Rpv + xhat_update(1);
%Ipv = (u - xhat(1))/Rpv;

%increase DC by .01:
DC = DC + .0001;
if(DC > 1)
    DC = 1;
end
Ac =[(-1/(Cpv*Rpv)) (-1/(Cpv)) (-DC/(Cpv)) 0 ;
    (1/(L1+L2) + L2*DC/(L1*(L1+L2)))  (-RL1/(L1+L2) -RL1*L2*DC/(L1*(L1+L2)))  (-RL2/(L1+L2) + RL2*DC/(L1+L2)) (-1/(L1+L2) + DC/(L1+L2));
    (1/(L1+L2) + L1*DC/(L2*(L1+L2)))  (-RL1/(L1+L2) + RL1*DC/(L1+L2)) (-RL2/(L1+L2)-RL2*L1*DC/(L2*(L1+L2))) (-1/(L1+L2) + DC/(L1+L2));
    0 0 (1/(Cout) - DC/(Cout)) (-1/(Rout*Cout))];
Aol_increase = eye(4) + Ac*Ts;
%predict 1 timestep ahead on
xhat_plus_on = Aol_increase*xhat_update + Bol*u;
Ipv_plus_on = (u - xhat_plus_on(1))/Rpv;
%decrease DC by .01
DC = DC - 2*.0001;
if(DC < 0) 
    DC = 0; end
Ac =[(-1/(Cpv*Rpv)) (-1/(Cpv)) (-DC/(Cpv)) 0 ;
    (1/(L1+L2) + L2*DC/(L1*(L1+L2)))  (-RL1/(L1+L2) -RL1*L2*DC/(L1*(L1+L2)))  (-RL2/(L1+L2) + RL2*DC/(L1+L2)) (-1/(L1+L2) + DC/(L1+L2));
    (1/(L1+L2) + L1*DC/(L2*(L1+L2)))  (-RL1/(L1+L2) + RL1*DC/(L1+L2)) (-RL2/(L1+L2)-RL2*L1*DC/(L2*(L1+L2))) (-1/(L1+L2) + DC/(L1+L2));
    0 0 (1/(Cout) - DC/(Cout)) (-1/(Rout*Cout))];
DC = DC + .0001;
Aol_decrease = eye(4) + Ac*Ts;
%predict 1 timestep ahead off
xhat_plus_off = Aol_decrease*xhat_update + Bol*u;
Ipv_plus_off = (u - xhat_plus_off(1))/Rpv;





%update function output and variables
P_t_1 = P_update;
xhat_t_1 = xhat_update;
xhat = xhat_update;


%%%%%%%%%%%%%%%%%%%%%%%%%%%%%%%
if (Ipv > 10)
    Ipv = 1;
end

Vpv = u;

persistent Vpv_t_1; %previous Vpv Sample
if isempty(Vpv_t_1)
    Vpv_t_1 = 0;
end
persistent Ipv_t_1; %previous Ipv Sample
if isempty(Ipv_t_1)
    Ipv_t_1 = 0;
end
persistent Dpv_t_1; % Iref (output) value from what is now 2 timesteps ago
if isempty(Dpv_t_1)
    Dpv_t_1 = 0;
end
persistent Dpv;  %Previous / Most recent Iref (output) Calc
if isempty(Dpv)
    Dpv = 0;
end

Ts = 15e-6; %sample rate
L = 3e-3; %inductance


delta_V = Vpv - Vpv_t_1;
delta_I = Ipv - Ipv_t_1;
delta_D = Dpv - Dpv_t_1;


%fixed vs adaptive
scale_factor_C = 10; %increase for larger output increments/swings
 Z =.001; %fixed 
%Z = scale_factor_C * abs(delta_I * delta_D); %adaptive

% custom adaptive to fix issues with no change causing 0 step size
 adapZ = scale_factor_C * abs(delta_I * delta_D);
% if(adapZ > .1)
%     Z = .1;
% elseif(adapZ > .001)
%     Z = adapZ;
% else
%     Z = .001;
% end

Ipred_1 = Ipv_plus_on;
Ipred_0 = Ipv_plus_off;
%Ipred_1 = Ipv + 2*(Ts/L) * Vpv; %MPC prediction for switch = 1
%Ipred_0 = Ipv + (Ts/(2*L)* (Vpv - Vout)); %MPC prediction for switch = 0 

if delta_V == 0 %Inc. Cond. Algo to determine Iref
    if delta_I == 0 
        Iref = Dpv; choice = 0;
    else
        if delta_I > 0
            Iref = Dpv - Z; choice = 1;
        else
            Iref = Dpv + Z; choice = 2;
        end
    end
else
    if (Ipv + (delta_I/delta_V) * Vpv) == 0
        Iref = Dpv; choice = 3;
    else
        if (Ipv + (delta_I/delta_V) * Vpv) > 0
            Iref = Dpv - Z; choice = 4;
        else
            Iref = Dpv + Z; choice = 5;
        end
    end
end

G1 = abs(Iref - Ipred_1); %Optimize MPC by applying Iref
G0 = abs(Iref - Ipred_0);
if G1 < G0
    DC = DC + .0001;
else
    DC = DC - .0001;
end

if (DC < 0)
    DC = 0;
end
if (DC > 1)
    DC = 1;
end

if (Iref < 0)
    Iref = .001;
end
%test = Ipv + (delta_I/delta_V) * Vpv;
test =  delta_V;
%update static variables here:
Vpv_t_1 = Vpv; %previous Vpv Sample
Ipv_t_1 = Ipv; %previous Ipv Sample
Dpv_t_1 = Dpv; % Iref (output) value from what is now 2 timesteps ago
Dpv = Iref;  %Previous / Most recent Iref (output) Calc

y = DC;

%debug purposes:
debug1 = Iref;
debug2 = delta_I/delta_V;

== matlab function project_589/MATLAB Function1 ==
  settings: updateMethod=DISCRETE
  data: u input; xhat output; y input; debug output
function [xhat, debug] = fcn(u, y)

X=u(1:4);
Vpv=u(5);
u=u(6);

y=(y);



persistent xhat_t_1; %previous xhat Sample
if isempty(xhat_t_1)
    xhat_t_1 = [.1; .1; .1; .1];
end

persistent P_t_1;
if isempty(P_t_1)
    P_t_1 = [.1 .1 .1 .1;
            .1 .1 .1 .1;
            .1 .1 .1 .1;
            .1 .1 .1 .1];
end


Cpv=260e-6;
Cout=260e-6;
L1=3e-3;
L2=3e-3;
Rout=100;
Rpv = 1;
RL1 = 1;
RL2 = 1;

% Compact form
A=[ -1/(Cpv*Rpv) -1/Cpv 0 0 ;
    1/(L1+L2) -RL1/(L1+L2) -RL2/(L1+L2) -1/(L1+L2) ;
    1/(L1+L2) -RL1/(L1+L2)  -RL2/(L1+L2) -1/(L1+L2);
    0 0 1/Cout -1/(Rout*Cout)];

B=[0 0 -1/(Cpv) 0;
    L2/(L1*(L1+L2)) -RL1*L2/(L1*(L1+L2)) RL2/(L1+L2) 1/(L1+L2);
     L1/(L2*(L1+L2)) RL1/(L1+L2) -RL2*L1/(L2*(L1+L2)) 1/(L1+L2);
    0  0 -1/(Cout) 0 ];
     
b=[0; 0; 0; 0];

d=[Vpv/(Cpv*Rpv); 0; 0; 0];


u_e = u;
F =[(-1/(Cpv*Rpv)) (-1/(Cpv)) (-u_e/(Cpv)) 0 ;
    (1/(L1+L2) + L2*u_e/(L1*(L1+L2)))  (-RL1/(L1+L2) -RL1*L2*u_e/(L1*(L1+L2)))  (-RL2/(L1+L2) + RL2*u_e/(L1+L2)) (-1/(L1+L2) + u_e/(L1+L2));
    (1/(L1+L2) + L1*u_e/(L2*(L1+L2)))  (-RL1/(L1+L2) + RL1*u_e/(L1+L2)) (-RL2/(L1+L2)-RL2*L1*u_e/(L2*(L1+L2))) (-1/(L1+L2) + u_e/(L1+L2));
    0 0 (1/(Cout) - u_e/(Cout)) (-1/(Rout*Cout))];

H = [0 0 0 1];

Q = [.000001 .000001 .000001 .000001;
    .000001 .000001 .000001 .000001;
    .000001 .000001 .000001 .000001;
    .000001 .000001 .000001 .000001];

R = .000001;

%prediction stage
xhat_pred = A*xhat_t_1+(B*xhat_t_1+b)*u+d;
P_pred = F*P_t_1*transpose(F)+ Q;

%update stage
y_update = y - H*xhat_pred;
S_update = H*P_pred*transpose(H) + R;
K_update = P_pred*transpose(H)*(1/S_update);
xhat_update = xhat_pred + K_update*y_update;
P_update = (eye(4) - K_update*H)*P_pred;


%update function output and variables
P_t_1 = P_update;
xhat_t_1 = xhat_update;
xhat = xhat_update;

== matlab function project_589/MATLAB Function ==
  settings: updateMethod=DISCRETE
  data: choice output; debug1 output; debug2 output; debug3 output; u input; y output
function [choice, debug1, debug2,debug3, y]= fcn(u)
Vpv=u(1);
Ipv=u(2);
Vout=u(3);

%This module contains the MPC-MPPT Control Algorithm

%The MPC module follows the flow chart of Fig. 8 in Referenced Research Paper

%This MATLAB fn block's settings have been changed to have a sampling rate
%of 15uS instead of being continous sample mode


%prevent crazy simulation transients from breaking the algorithm:
if (Ipv > 10)
    Ipv = 1;
end

persistent Vpv_t_1; %previous Vpv Sample
if isempty(Vpv_t_1)
    Vpv_t_1 = 0;
end
persistent Ipv_t_1; %previous Ipv Sample
if isempty(Ipv_t_1)
    Ipv_t_1 = 0;
end
persistent Dpv_t_1; % Iref (output) value from what is now 2 timesteps ago
if isempty(Dpv_t_1)
    Dpv_t_1 = 0;
end
persistent Dpv;  %Previous / Most recent Iref (output) Calc
if isempty(Dpv)
    Dpv = 0;
end

Ts = 15e-6; %sample rate
L = 3e-3; %inductance

Power = Vpv * Ipv;
delta_P = Power - (Vpv_t_1 * Ipv_t_1);
delta_V = Vpv - Vpv_t_1;
delta_I = Ipv - Ipv_t_1;
delta_D = Dpv - Dpv_t_1;


%fixed vs adaptive
S = .001;
M = 10;
Z =.001;%delta_P/delta_V * exp(-M*Dpv); %.0005; %fixed 
%Z = scale_factor_C * abs(delta_I * delta_D); %adaptive

% custom adaptive to fix issues with no change causing 0 step size
 %adapZ = scale_factor_C * abs(delta_I * delta_D);
% if(adapZ > .1)
%     Z = .1;
% elseif(adapZ > .001)
%     Z = adapZ;
% else
%     Z = .001;
% end


Ipred_1 = Ipv + 2*(Ts/L) * Vpv; %MPC prediction for switch = 1
Ipred_0 = Ipv + (Ts/(2*L)* (Vpv - Vout)); %MPC prediction for switch = 0 

if delta_V == 0 %Inc. Cond. Algo to determin Iref
    if delta_I == 0 
        Iref = Dpv; choice = 0;
    else
        if delta_I > 0
            Iref = Dpv - Z; choice = 1;
        else
            Iref = Dpv + Z; choice = 2;
        end
    end
else
    if (Ipv + (delta_I/delta_V) * Vpv) == 0
        Iref = Dpv; choice = 3;
    else
        if (Ipv + (delta_I/delta_V) * Vpv) > 0
            Iref = Dpv - Z; choice = 4;
        else
            Iref = Dpv + Z; choice = 5;
        end
    end
end

G1 = abs(Iref - Ipred_1); %Optimize MPC by applying Iref
G0 = abs(Iref - Ipred_0);
if G1 < G0
    y = 1;
else
    y = 0;
end

if (Iref < 0)
    Iref = .001;
end
%test = Ipv + (delta_I/delta_V) * Vpv;
test =  delta_V;
%update static variables here:
Vpv_t_1 = Vpv; %previous Vpv Sample
Ipv_t_1 = Ipv; %previous Ipv Sample
Dpv_t_1 = Dpv; % Iref (output) value from what is now 2 timesteps ago
Dpv = Iref;  %Previous / Most recent Iref (output) Calc

%debug purposes:
debug1 = Ipred_1;
debug2 = Ipred_0;
debug3 = Iref;

== matlab function project_589/MATLAB Function2 ==
  settings: updateMethod=DISCRETE
  data: Y output; u input
function Y = fcn(u)

persistent D; 
if isempty(D)
    D = 0;
end

persistent T_on; 
if isempty(T_on)
    T_on = 0;
end

persistent T_off; 
if isempty(T_off)
    T_off = 0;
end

persistent u_prev; 
if isempty(u_prev)
    u_prev = 0;
end

persistent Ts; 
if isempty(Ts)
    Ts = 0;
end



if(u_prev == 0 && u == 1)
    D = T_on / Ts;
    Ts = 15e-6;
    T_on = 15e-6;
    T_off = 0;
else
    D = D;
    if(u == 1)
    Ts = Ts + 15e-6;
    T_on = T_on + 15e-6;
    else
     Ts = Ts + 15e-6;
     T_off = T_off + 15e-6;
    end
end

%prevent holding the output to break the system
if(Ts > 19*15e-6)
    if(u == 1) D = 1;
    else D = 0;
    end
end

u_prev = u;
Y = D;

== matlab function project_589/MATLAB Function3 ==
  data: u input; y output
function y = fcn(u)

X=u(1:4);
Vpv=u(5);
u=u(6);


%5/10/2021 UPDATED
% parameters:


Cpv=260e-6;
Cout=260e-6;
L1=3e-3;
L2=3e-3;
Rout=100;
Rpv = 1;
RL1 = 1;
RL2 = 1;

% Compact form
A=[ -1/(Cpv*Rpv) -1/Cpv 0 0 ;
    1/(L1+L2) -RL1/(L1+L2) -RL2/(L1+L2) -1/(L1+L2) ;
    1/(L1+L2) -RL1/(L1+L2)  -RL2/(L1+L2) -1/(L1+L2);
    0 0 1/Cout -1/(Rout*Cout)];

B=[0 0 -1/(Cpv) 0;
    L2/(L1*(L1+L2)) -RL1*L2/(L1*(L1+L2)) RL2/(L1+L2) 1/(L1+L2);
     L1/(L2*(L1+L2)) RL1/(L1+L2) -RL2*L1/(L2*(L1+L2)) 1/(L1+L2);
    0  0 -1/(Cout) 0 ];
     
     
b=[0; 0; 0; 0];

d=[Vpv/(Cpv*Rpv); 0; 0; 0];

y = A*X+(B*X+b)*u+d;

== matlab function project_589/MATLAB Function4 ==
  data: u input; y output
function y = fcn(u)

X=u(1:4);
Vpv=u(5);
u=u(6);



% parameters:
%5/10/2021 u_ePDATED


Cpv=260e-6;
Cout=260e-6;
L1=3e-3;
L2=3e-3;
Rout=100;
Rpv = 1;
RL1 = 1;
RL2 = 1;

u_e = .5;

% Compact form
A=[(-1/(Cpv*Rpv)) (-1/(Cpv)) (-u_e/(Cpv)) 0 ;
    (1/(L1+L2) + L2*u_e/(L1*(L1+L2)))  (-RL1/(L1+L2) -RL1*L2*u_e/(L1*(L1+L2)))  (-RL2/(L1+L2) + RL2*u_e/(L1+L2)) (-1/(L1+L2) + u_e/(L1+L2));
    (1/(L1+L2) + L1*u_e/(L2*(L1+L2)))  (-RL1/(L1+L2) + RL1*u_e/(L1+L2)) (-RL2/(L1+L2)-RL2*L1*u_e/(L2*(L1+L2))) (-1/(L1+L2) + u_e/(L1+L2));
    0 0 (1/(Cout) - u_e/(Cout)) (-1/(Rout*Cout))];

%VCpv = (L2*RL1*Rout*Vpv*u_e^2 - 2*L2*RL1*Rout*Vpv*u_e + L1*RL1*RL2*Vpv + L2*RL1*RL2*Vpv + L2*RL1*Rout*Vpv)/(L1*RL1*RL2 + L2*RL1*RL2 + L2*RL1*Rout + L2*RL2*Rpv - L1*Rout*Rpv + L2*Rout*Rpv + L2*RL1*Rout*u_e^2 + L2*RL1*Rpv*u_e^2 - L1*Rout*Rpv*u_e^2 + L2*Rout*Rpv*u_e^2 - 2*L2*RL1*Rout*u_e + L1*RL1*Rpv*u_e + L1*RL2*Rpv*u_e + 2*L1*Rout*Rpv*u_e - 2*L2*Rout*Rpv*u_e);
%IL1 = (Vpv*(L2*RL2 - L1*Rout + L2*Rout + L1*RL2*u_e + 2*L1*Rout*u_e - 2*L2*Rout*u_e - L1*Rout*u_e^2 + L2*Rout*u_e^2))/(L1*RL1*RL2 + L2*RL1*RL2 + L2*RL1*Rout + L2*RL2*Rpv - L1*Rout*Rpv + L2*Rout*Rpv + L2*RL1*Rout*u_e^2 + L2*RL1*Rpv*u_e^2 - L1*Rout*Rpv*u_e^2 + L2*Rout*Rpv*u_e^2 - 2*L2*RL1*Rout*u_e + L1*RL1*Rpv*u_e + L1*RL2*Rpv*u_e + 2*L1*Rout*Rpv*u_e - 2*L2*Rout*Rpv*u_e);
%IL2 = (RL1*Vpv*(L1 + L2*u_e))/(L1*RL1*RL2 + L2*RL1*RL2 + L2*RL1*Rout + L2*RL2*Rpv - L1*Rout*Rpv + L2*Rout*Rpv + L2*RL1*Rout*u_e^2 + L2*RL1*Rpv*u_e^2 - L1*Rout*Rpv*u_e^2 + L2*Rout*Rpv*u_e^2 - 2*L2*RL1*Rout*u_e + L1*RL1*Rpv*u_e + L1*RL2*Rpv*u_e + 2*L1*Rout*Rpv*u_e - 2*L2*Rout*Rpv*u_e);
%VCout = -(RL1*Rout*Vpv*(L1 + L2*u_e)*(u_e - 1))/(L1*RL1*RL2 + L2*RL1*RL2 + L2*RL1*Rout + L2*RL2*Rpv - L1*Rout*Rpv + L2*Rout*Rpv + L2*RL1*Rout*u_e^2 + L2*RL1*Rpv*u_e^2 - L1*Rout*Rpv*u_e^2 + L2*Rout*Rpv*u_e^2 - 2*L2*RL1*Rout*u_e + L1*RL1*Rpv*u_e + L1*RL2*Rpv*u_e + 2*L1*Rout*Rpv*u_e - 2*L2*Rout*Rpv*u_e);

VCpv = (L2*RL1*Rout*Vpv*u_e^2 - 2*L2*RL1*Rout*Vpv*u_e + L1*RL1*RL2*Vpv + L2*RL1*RL2*Vpv + L2*RL1*Rout*Vpv)/(L1*RL1*RL2 + L2*RL1*RL2 + L2*RL1*Rout + L2*RL2*Rpv - L1*Rout*Rpv + L2*Rout*Rpv + L2*RL1*Rout*u_e^2 + L2*RL1*Rpv*u_e^2 - L1*Rout*Rpv*u_e^2 + L2*Rout*Rpv*u_e^2 - 2*L2*RL1*Rout*u_e + L1*RL1*Rpv*u_e + L1*RL2*Rpv*u_e + 2*L1*Rout*Rpv*u_e - 2*L2*Rout*Rpv*u_e);
IL1 = (Vpv*(L2*RL2 - L1*Rout + L2*Rout + L1*RL2*u_e + 2*L1*Rout*u_e - 2*L2*Rout*u_e - L1*Rout*u_e^2 + L2*Rout*u_e^2))/(L1*RL1*RL2 + L2*RL1*RL2 + L2*RL1*Rout + L2*RL2*Rpv - L1*Rout*Rpv + L2*Rout*Rpv + L2*RL1*Rout*u_e^2 + L2*RL1*Rpv*u_e^2 - L1*Rout*Rpv*u_e^2 + L2*Rout*Rpv*u_e^2 - 2*L2*RL1*Rout*u_e + L1*RL1*Rpv*u_e + L1*RL2*Rpv*u_e + 2*L1*Rout*Rpv*u_e - 2*L2*Rout*Rpv*u_e);
IL2 =  (RL1*Vpv*(L1 + L2*u_e))/(L1*RL1*RL2 + L2*RL1*RL2 + L2*RL1*Rout + L2*RL2*Rpv - L1*Rout*Rpv + L2*Rout*Rpv + L2*RL1*Rout*u_e^2 + L2*RL1*Rpv*u_e^2 - L1*Rout*Rpv*u_e^2 + L2*Rout*Rpv*u_e^2 - 2*L2*RL1*Rout*u_e + L1*RL1*Rpv*u_e + L1*RL2*Rpv*u_e + 2*L1*Rout*Rpv*u_e - 2*L2*Rout*Rpv*u_e);
VCout =  -(RL1*Rout*Vpv*(L1 + L2*u_e)*(u_e - 1))/(L1*RL1*RL2 + L2*RL1*RL2 + L2*RL1*Rout + L2*RL2*Rpv - L1*Rout*Rpv + L2*Rout*Rpv + L2*RL1*Rout*u_e^2 + L2*RL1*Rpv*u_e^2 - L1*Rout*Rpv*u_e^2 + L2*Rout*Rpv*u_e^2 - 2*L2*RL1*Rout*u_e + L1*RL1*Rpv*u_e + L1*RL2*Rpv*u_e + 2*L1*Rout*Rpv*u_e - 2*L2*Rout*Rpv*u_e);
 
% B=[ -IL2/Cpv;
%     L2*VCpv/(L1*(L1+L2))-RL1*L2*IL1/(L1*(L1+L2))+RL2*IL2/(L1+L2)+VCout/(L1+L2);
%     L1*VCpv/(L2*(L1+L2))+RL1*IL1/(L1+L2)-RL2*L1*IL2/(L2*(L1+L2))+VCout/(L1+L2);
%      -IL2/Cout];


B = [1/(Cpv*Rpv);
    0;
    0;
    0];

u = Vpv;

y = A*X+B*u;

== matlab function project_589/MATLAB Function5 ==
  data: D input; xhat output; u_Vpv input; Vout input; Ipv output; Ipv_plus_on output; Ipv_plus_off output
function [xhat, Ipv, Ipv_plus_on, Ipv_plus_off]  = fcn(D,u_Vpv, Vout)
%Kalman filter design using Small Signal Model of Circuit

%The purpose of this module is to approximate Ipv and Vpv so that a sensor
%is not needed for those variables, it also functions to remove noise and
%could possibly replace the MCP module using its own predictions

%Existing Model assumes Constant Vpv with added series resistor so that
% Ipv = (Vpv - Vcpv)/Rpv
%Also assumes L1 = L2

%Existing state variables: IL1 IL2 Vo Vcpv

%define circuit parameters 

Cpv=260e-6;
Cout=260e-6;
L1=3e-3;
L2=3e-3;
Rout=100;
Rpv = 1;
RL1 = 1;
RL2 = 1;

u_e = D;
y = Vout;
u = u_Vpv;

Ts = 15e-6;
% Continuous Time Small Signal State Space
%Aol = [0.943784461257301,-0.0559330122345799,-0.0279395312339836,5.29606701473712e-05;0.00363447688363775,0.996152021590196,-0.00131615408875196,-0.00124644633684318;0.00363447688363775,-0.00135110080726459,0.996186968308708,-0.00124644633684318;5.29606701473712e-05,-1.90030480999995e-05,0.0287831492829427,0.999405251934562];
Ac =[(-1/(Cpv*Rpv)) (-1/(Cpv)) (-u_e/(Cpv)) 0 ;
    (1/(L1+L2) + L2*u_e/(L1*(L1+L2)))  (-RL1/(L1+L2) -RL1*L2*u_e/(L1*(L1+L2)))  (-RL2/(L1+L2) + RL2*u_e/(L1+L2)) (-1/(L1+L2) + u_e/(L1+L2));
    (1/(L1+L2) + L1*u_e/(L2*(L1+L2)))  (-RL1/(L1+L2) + RL1*u_e/(L1+L2)) (-RL2/(L1+L2)-RL2*L1*u_e/(L2*(L1+L2))) (-1/(L1+L2) + u_e/(L1+L2));
    0 0 (1/(Cout) - u_e/(Cout)) (-1/(Rout*Cout))];
Bc = [1/(Cpv*Rpv);
    0;
    0;
    0];
 Cc = [0 0 0 1];
 
 Dc = zeros(size(Cc,1), size(Bc,2));
 
 %discretize my state space model using ZOH method
 Aol = eye(4) + Ac*Ts;
 Bol = Bc*Ts;
 Col = Cc;
 Dol = Dc;
 
 
%Bol = [0.0560566260169120;0.000105941817191590;0.000105941817191590;1.02384484238660e-06];

%Col = [0,0,0,1];

%Dol = 0;
 %Design the Observer System:
 

 %covar matricies, process q, measurement r -- must be positive numbers
 Qcov = diag(.000001*ones(1,4)); %modify the numbers to change how it filters noise
 Rcov = diag(.000001*ones(1,1)); %modify the numbers to change how it filters noise
 

persistent xhat_t_1; %previous xhat Sample
if isempty(xhat_t_1)
    xhat_t_1 = [.1; .1; .1; .1];
end

persistent P_t_1;
if isempty(P_t_1)
    P_t_1 = [.1 .1 .1 .1;
            .1 .1 .1 .1;
            .1 .1 .1 .1;
            .1 .1 .1 .1];
end


%prediction stage
xhat_pred = Aol*xhat_t_1+Bol*u;
P_pred = Aol*P_t_1*transpose(Aol)+ Qcov;

%update stage
y_update = y - Col*xhat_pred;
S_update = Col*P_pred*transpose(Col) + Rcov;
K_update = P_pred*transpose(Col)*(1/S_update);
xhat_update = xhat_pred + K_update*y_update;
P_update = (eye(4) - K_update*Col)*P_pred;


%increase DC by .01:
u_e = u_e + .0005;
if(u_e > 1)
    u_e = 1;
end
Ac =[(-1/(Cpv*Rpv)) (-1/(Cpv)) (-u_e/(Cpv)) 0 ;
    (1/(L1+L2) + L2*u_e/(L1*(L1+L2)))  (-RL1/(L1+L2) -RL1*L2*u_e/(L1*(L1+L2)))  (-RL2/(L1+L2) + RL2*u_e/(L1+L2)) (-1/(L1+L2) + u_e/(L1+L2));
    (1/(L1+L2) + L1*u_e/(L2*(L1+L2)))  (-RL1/(L1+L2) + RL1*u_e/(L1+L2)) (-RL2/(L1+L2)-RL2*L1*u_e/(L2*(L1+L2))) (-1/(L1+L2) + u_e/(L1+L2));
    0 0 (1/(Cout) - u_e/(Cout)) (-1/(Rout*Cout))];
Aol_increase = eye(4) + Ac*Ts;
%predict 1 timestep ahead on
xhat_plus_on = Aol_increase*xhat_update + Bol*u;
Ipv_plus_on = (u - xhat_plus_on(1))/Rpv;
%decrease DC by .01
u_e = u_e - 2*.0005;
if(u_e < 0) 
    u_e = 0; end
Ac =[(-1/(Cpv*Rpv)) (-1/(Cpv)) (-u_e/(Cpv)) 0 ;
    (1/(L1+L2) + L2*u_e/(L1*(L1+L2)))  (-RL1/(L1+L2) -RL1*L2*u_e/(L1*(L1+L2)))  (-RL2/(L1+L2) + RL2*u_e/(L1+L2)) (-1/(L1+L2) + u_e/(L1+L2));
    (1/(L1+L2) + L1*u_e/(L2*(L1+L2)))  (-RL1/(L1+L2) + RL1*u_e/(L1+L2)) (-RL2/(L1+L2)-RL2*L1*u_e/(L2*(L1+L2))) (-1/(L1+L2) + u_e/(L1+L2));
    0 0 (1/(Cout) - u_e/(Cout)) (-1/(Rout*Cout))];

Aol_decrease = eye(4) + Ac*Ts;
%predict 1 timestep ahead off
xhat_plus_off = Aol_decrease*xhat_update + Bol*u;
Ipv_plus_off = (u - xhat_plus_off(1))/Rpv;

%update function output and variables
P_t_1 = P_update;
xhat_t_1 = xhat_update;
xhat = xhat_update;
Ipv = (u - xhat(1))/Rpv;
